simulink model "Task1"  (R2013b)
settings: Solver=ode45  StartTime=0.0  StopTime=1  RelTol=1e-3
settings Model: Creator=barnetdavi  LastModifiedBy=barnetdavi

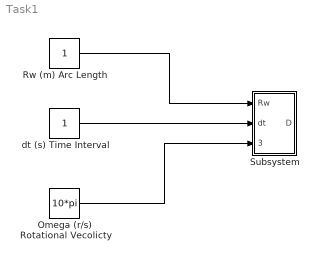
== system Task1 ==
  "Omega (r/s) Rotational Vecolicty " : Constant  Value=10*pi
  Rw (m) Arc Length : Constant
  Subsystem : Subsystem
  dt (s) Time Interval : Constant
  wires:
  Rw (m) Arc Length/1 -> Subsystem/1(Rw)
  dt (s) Time Interval/1 -> Subsystem/2(dt)
  "Omega (r/s) Rotational Vecolicty "/1 -> Subsystem/3(Omega)

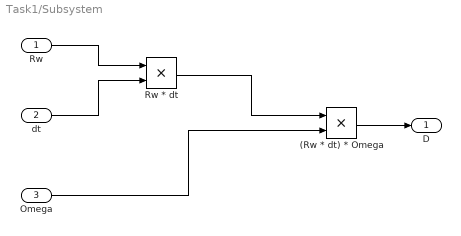
== system Task1/Subsystem ==
  Rw : Inport
  dt : Inport  Port=2
  Omega : Inport  Port=3
  (Rw * dt) * Omega : Product
  Rw * dt : Product
  D : Outport
  wires:
  dt/1 -> Rw * dt/2
  Rw/1 -> Rw * dt/1
  (Rw * dt) * Omega/1 -> D/1
  Omega/1 -> (Rw * dt) * Omega/2
  Rw * dt/1 -> (Rw * dt) * Omega/1
